simulink model "testsim"  (R2019a)
settings: Solver=VariableStepAuto  StartTime=0.0  StopTime=13  RelTol=1e-3
settings Model: Creator=owl06  LastModifiedBy=owl06

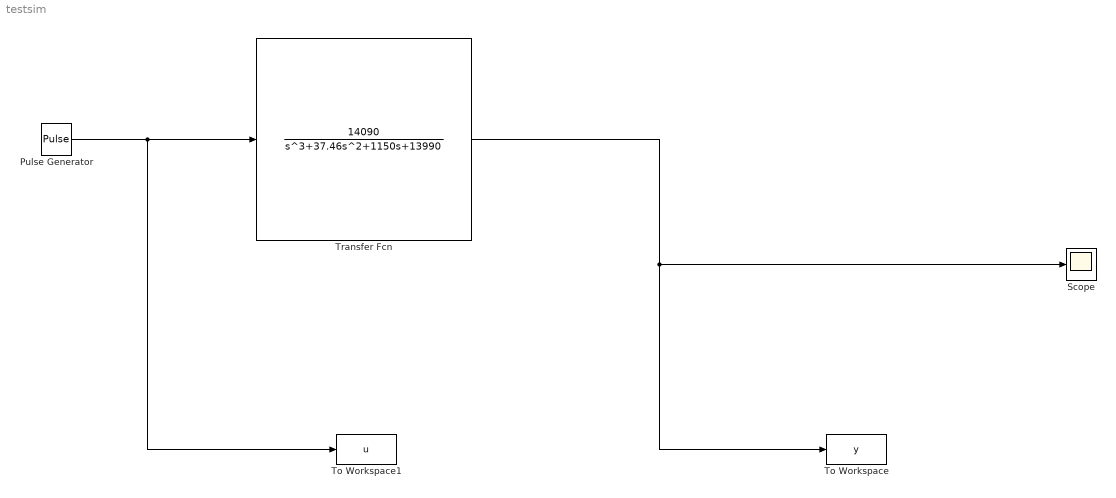
== system testsim ==
  Pulse Generator : DiscretePulseGenerator  PulseType=Time based  Amplitude=8.3  Period=4  PulseWidth=50  PhaseDelay=2
  Scope : Scope
  To Workspace : ToWorkspace  VariableName=y  SaveFormat=Structure With Time  SampleTime=0.001
  To Workspace1 : ToWorkspace  VariableName=u  SaveFormat=Structure With Time  SampleTime=0.001
  Transfer Fcn : TransferFcn  Numerator=[14090]  Denominator=[1 37.46 1150 13990]
  wires:
  Pulse Generator/1 -> To Workspace1/1, Transfer Fcn/1
  Transfer Fcn/1 -> Scope/1, To Workspace/1
